simulink model "Feeder"  (R2016b)
settings: Solver=ode1  StartTime=0.0  StopTime=inf  FixedStep=Ts  RelTol=1e-3
values from neighbouring files (symbols this model uses):
  clk = ~clk    [AC_Feeder_Control_Param.m]    (also in AC_Feeder_Control_Param_02-CORPGYEGTI03-P.m = logical(0); AC_Feeder_Control_Param_02.m = logical(0); Feeder_Param.m)
  r = randi(100)    [Feeder_Param.m]
settings Model: Creator=sixifo  LastModifiedBy=sixifo

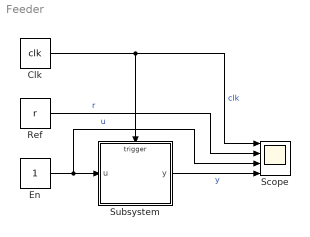
== system Feeder ==
  Clk : Constant  Value=clk
  En : Constant
  Ref : Constant  Value=r
  Scope : Scope  NumInputPorts=4
  Subsystem : Subsystem
  wires:
  En/1 -> Scope/3, Subsystem/1(u)  "u"
  Ref/1 -> Scope/2  "r"
  Subsystem/1(y) -> Scope/4  "y"
  Clk/1 -> Scope/1, Subsystem/Trigger  "clk"

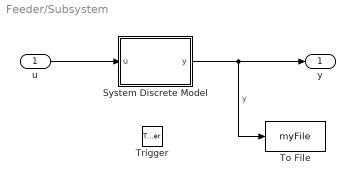
== system Feeder/Subsystem ==
  u : Inport
  Trigger : TriggerPort  VariantControl=Variant  PortDimensions=1
  System Discrete Model : MATLAB Function  TreatAsAtomicUnit=on
  To File : ToFile  Filename=myFile  MatrixName=yo
  y : Outport
  wires:
  u/1 -> System Discrete Model/1(u)
  System Discrete Model/1(y) -> To File/1, y/1  "y"

== matlab function Feeder/Subsystem/System Discrete Model ==
  data: u input; y output
function y = fcn(u)

y=u*rand*100; % Load variable stored in .mat File
